simulink model "Gate_Harness"  (R2022b)
settings: Solver=VariableStepAuto  StartTime=0.0  StopTime=80.0  RelTol=1e-3
(part 2 of 2)

== stateflow chart Gate_Harness/Test Sequence ==
  settings: updateMethod=DISCRETE  sampleTime=0.2
  state Apertura_Chiusura_con_B1
    state INIT
      %% Initialize data outputs.
      p1 = true;
      p2 = false;
      start = false;
      b1 = false;
      b2 = false;
      b3 = false;
      verify(enable_green == false);
      verify(enable_yellow == false);
      verify(enable_red == false);
      verify(blink_green == false);
      verify(blink_yellow == false);
    state TURN_ON
      start = true;
    state CLOSE
      verify(enable_green == false);
      verify(enable_yellow == false);
      verify(enable_red == false);
      verify(blink_green == false);
      verify(blink_yellow == false);
    state PRESSED
      b1 = true;
    state RELEASED_BUTTON
      b1 = false;
    state OPENING_GATE
      p2 = true;
      verify(enable_green == false);
      verify(enable_yellow == false);
      verify(enable_red == false);
      verify(blink_green == false);
      verify(blink_yellow == true);
    state OPEN_GATE
      verify(enable_green == true);
      verify(enable_yellow == true);
      verify(enable_red == true);
      verify(blink_green == false);
      verify(blink_yellow == false);
    state PRESSED_AGAIN
      b1 = true;
    state RELEASED_BUTTON_AGAIN
      b1 = false;
    state CLOSING_GATE
      verify(enable_green == false);
      verify(enable_yellow == false);
      verify(enable_red == false);
      verify(blink_green == false);
      verify(blink_yellow == true);
    state ACTIVATE_P2
      p2 = false;
    state CLOSE_GATE
      verify(enable_green == false);
      verify(enable_yellow == false);
      verify(enable_red == false);
      verify(blink_green == false);
      verify(blink_yellow == false);
    state FINAL
    (default) -> Apertura_Chiusura_con_B1.INIT
    Apertura_Chiusura_con_B1.INIT -> Apertura_Chiusura_con_B1.TURN_ON : [
        | after(2, sec)
        | ]
    Apertura_Chiusura_con_B1.TURN_ON -> Apertura_Chiusura_con_B1.CLOSE : [
        | after(3, sec)
        | ]
    Apertura_Chiusura_con_B1.CLOSE -> Apertura_Chiusura_con_B1.PRESSED : [
        | after(2, sec)
        | ]
    Apertura_Chiusura_con_B1.PRESSED -> Apertura_Chiusura_con_B1.RELEASED_BUTTON : [
        | after(2, sec)
        | ]
    Apertura_Chiusura_con_B1.RELEASED_BUTTON -> Apertura_Chiusura_con_B1.OPENING_GATE : [
        | after(0.4, sec)
        | ]
    Apertura_Chiusura_con_B1.OPENING_GATE -> Apertura_Chiusura_con_B1.OPEN_GATE : [
        | after(10, sec)
        | ]
    Apertura_Chiusura_con_B1.OPEN_GATE -> Apertura_Chiusura_con_B1.PRESSED_AGAIN : [
        | after(4, sec)
        | ]
    Apertura_Chiusura_con_B1.PRESSED_AGAIN -> Apertura_Chiusura_con_B1.RELEASED_BUTTON_AGAIN : [
        | after(2, sec)
        | ]
    Apertura_Chiusura_con_B1.RELEASED_BUTTON_AGAIN -> Apertura_Chiusura_con_B1.CLOSING_GATE : [
        | after(0.4, sec)
        | ]
    Apertura_Chiusura_con_B1.CLOSING_GATE -> Apertura_Chiusura_con_B1.ACTIVATE_P2 : [
        | after(9.4, sec)
        | ]
    Apertura_Chiusura_con_B1.ACTIVATE_P2 -> Apertura_Chiusura_con_B1.CLOSE_GATE : [
        | after(1, sec)
        | ]
    Apertura_Chiusura_con_B1.CLOSE_GATE -> Apertura_Chiusura_con_B1.FINAL : [
        | after(6, sec)
        | ]
  state Chiusura_Automatica
    state INIT
      %% Initialize data outputs.
      p1 = true;
      p2 = false;
      start = false;
      b1 = false;
      b2 = false;
      b3 = false;
      verify(enable_green == false);
      verify(enable_yellow == false);
      verify(enable_red == false);
      verify(blink_green == false);
      verify(blink_yellow == false);
    state TURN_ON
      start = true;
    state CLOSE
      verify(enable_green == false);
      verify(enable_yellow == false);
      verify(enable_red == false);
      verify(blink_green == false);
      verify(blink_yellow == false);
    state PRESSED
      b1 = true;
    state RELEASED_BUTTON
      b1 = false;
    state OPENING_GATE
      p2 = true;
      verify(enable_green == false);
      verify(enable_yellow == false);
      verify(enable_red == false);
      verify(blink_green == false);
      verify(blink_yellow == true);
    state OPEN_GATE
      verify(enable_green == true);
      verify(enable_yellow == true);
      verify(enable_red == true);
      verify(blink_green == false);
      verify(blink_yellow == false);
    state CLOSING_GATE
      verify(enable_green == false);
      verify(enable_yellow == false);
      verify(enable_red == false);
      verify(blink_green == false);
      verify(blink_yellow == true);
    state ACTIVATE_P2
      p2 = false;
    state CLOSE_GATE
      verify(enable_green == false);
      verify(enable_yellow == false);
      verify(enable_red == false);
      verify(blink_green == false);
      verify(blink_yellow == false);
    state FINAL
    (default) -> Chiusura_Automatica.INIT
    Chiusura_Automatica.INIT -> Chiusura_Automatica.TURN_ON : [
        | after(2, sec)
        | ]
    Chiusura_Automatica.TURN_ON -> Chiusura_Automatica.CLOSE : [
        | after(3, sec)
        | ]
    Chiusura_Automatica.CLOSE -> Chiusura_Automatica.PRESSED : [
        | after(2, sec)
        | ]
    Chiusura_Automatica.PRESSED -> Chiusura_Automatica.RELEASED_BUTTON : [
        | after(2, sec)
        | ]
    Chiusura_Automatica.RELEASED_BUTTON -> Chiusura_Automatica.OPENING_GATE : [
        | after(0.4, sec)
        | ]
    Chiusura_Automatica.OPENING_GATE -> Chiusura_Automatica.OPEN_GATE : [
        | after(10, sec)
        | ]
    Chiusura_Automatica.OPEN_GATE -> Chiusura_Automatica.CLOSING_GATE : [
        | after(10, sec)
        | ]
    Chiusura_Automatica.CLOSING_GATE -> Chiusura_Automatica.ACTIVATE_P2 : [
        | after(9.4, sec)
        | ]
    Chiusura_Automatica.ACTIVATE_P2 -> Chiusura_Automatica.CLOSE_GATE : [
        | after(2, sec)
        | ]
    Chiusura_Automatica.CLOSE_GATE -> Chiusura_Automatica.FINAL : [
        | after(4, sec)
        | ]
  state Richiesta_Chiusura_durante_Apertura
    state INIT
      %% Initialize data outputs.
      p1 = true;
      p2 = false;
      start = false;
      b1 = false;
      b2 = false;
      b3 = false;
      verify(enable_green == false);
      verify(enable_yellow == false);
      verify(enable_red == false);
      verify(blink_green == false);
      verify(blink_yellow == false);
    state TURN_ON
      start = true;
    state CLOSE
      verify(enable_green == false);
      verify(enable_yellow == false);
      verify(enable_red == false);
      verify(blink_green == false);
      verify(blink_yellow == false);
    state PRESSED
      b1 = true;
    state RELEASED_BUTTON
      b1 = false;
    state OPENING_GATE
      p2 = true;
      verify(enable_green == false);
      verify(enable_yellow == false);
      verify(enable_red == false);
      verify(blink_green == false);
      verify(blink_yellow == true);
    state PRESSED_AGAIN
      b1 = true;
    state RELEASED_BUTTON_AGAIN
      b1 = false;
    state CLOSING_GATE
      verify(enable_green == false);
      verify(enable_yellow == false);
      verify(enable_red == false);
      verify(blink_green == false);
      verify(blink_yellow == true);
    state ACTIVATE_P2
      p2 = false;
    state CLOSE_GATE
      verify(enable_green == false);
      verify(enable_yellow == false);
      verify(enable_red == false);
      verify(blink_green == false);
      verify(blink_yellow == false);
    state FINAL
    (default) -> Richiesta_Chiusura_durante_Apertura.INIT
    Richiesta_Chiusura_durante_Apertura.INIT -> Richiesta_Chiusura_durante_Apertura.TURN_ON : [
        | after(2, sec)
        | ]
    Richiesta_Chiusura_durante_Apertura.TURN_ON -> Richiesta_Chiusura_durante_Apertura.CLOSE : [
        | after(3, sec)
        | ]
    Richiesta_Chiusura_durante_Apertura.CLOSE -> Richiesta_Chiusura_durante_Apertura.PRESSED : [
        | after(2, sec)
        | ]
    Richiesta_Chiusura_durante_Apertura.PRESSED -> Richiesta_Chiusura_durante_Apertura.RELEASED_BUTTON : [
        | after(2, sec)
        | ]
    Richiesta_Chiusura_durante_Apertura.RELEASED_BUTTON -> Richiesta_Chiusura_durante_Apertura.OPENING_GATE : [
        | after(0.4, sec)
        | ]
    Richiesta_Chiusura_durante_Apertura.OPENING_GATE -> Richiesta_Chiusura_durante_Apertura.PRESSED_AGAIN : [
        | after(3, sec)
        | ]
    Richiesta_Chiusura_durante_Apertura.PRESSED_AGAIN -> Richiesta_Chiusura_durante_Apertura.RELEASED_BUTTON_AGAIN : [
        | after(2, sec)
        | ]
    Richiesta_Chiusura_durante_Apertura.RELEASED_BUTTON_AGAIN -> Richiesta_Chiusura_durante_Apertura.CLOSING_GATE : [
        | after(0.4, sec)
        | ]
    Richiesta_Chiusura_durante_Apertura.CLOSING_GATE -> Richiesta_Chiusura_durante_Apertura.ACTIVATE_P2 : [
        | after(9.4, sec)
        | ]
    Richiesta_Chiusura_durante_Apertura.ACTIVATE_P2 -> Richiesta_Chiusura_durante_Apertura.CLOSE_GATE : [
        | after(1, sec)
        | ]
    Richiesta_Chiusura_durante_Apertura.CLOSE_GATE -> Richiesta_Chiusura_durante_Apertura.FINAL : [
        | after(6, sec)
        | ]
  state Richiesta_Apertura_durante_Chiusura
    state INIT
      %% Initialize data outputs.
      p1 = true;
      p2 = true;
      start = false;
      b1 = false;
      b2 = false;
      b3 = false;
      verify(enable_green == false);
      verify(enable_yellow == false);
      verify(enable_red == false);
      verify(blink_green == false);
      verify(blink_yellow == false);
    state TURN_ON
      start = true;
    state CLOSING_GATE
      verify(enable_green == false);
      verify(enable_yellow == false);
      verify(enable_red == false);
      verify(blink_green == false);
      verify(blink_yellow == true);
    state B1_PRESSED
      b1 = true;
    state B1_RELEASED
      b1 = false;
    state OPENING_GATE
      verify(enable_green == false);
      verify(enable_yellow == false);
      verify(enable_red == false);
      verify(blink_green == false);
      verify(blink_yellow == true);
    state FINAL
      start = false;
    (default) -> Richiesta_Apertura_durante_Chiusura.INIT
    Richiesta_Apertura_durante_Chiusura.INIT -> Richiesta_Apertura_durante_Chiusura.TURN_ON : [
        | after(2, sec)
        | ]
    Richiesta_Apertura_durante_Chiusura.CLOSING_GATE -> Richiesta_Apertura_durante_Chiusura.B1_PRESSED : [
        | after(4, sec)
        | ]
    Richiesta_Apertura_durante_Chiusura.B1_PRESSED -> Richiesta_Apertura_durante_Chiusura.B1_RELEASED : [
        | after(2, sec)
        | ]
    Richiesta_Apertura_durante_Chiusura.B1_RELEASED -> Richiesta_Apertura_durante_Chiusura.OPENING_GATE : [
        | after(0.4, sec)
        | ]
    Richiesta_Apertura_durante_Chiusura.OPENING_GATE -> Richiesta_Apertura_durante_Chiusura.FINAL : [
        | after(4, sec)
        | ]
    Richiesta_Apertura_durante_Chiusura.TURN_ON -> Richiesta_Apertura_durante_Chiusura.CLOSING_GATE : [
        | after(3, sec)
        | ]
  state Incremento_Tempo_Lavoro
    state INIT
      %% Initialize data outputs.
      p1 = true;
      p2 = false;
      start = false;
      b1 = false;
      b2 = false;
      b3 = false;
      n = 0;
      verify(enable_green == false);
      verify(enable_yellow == false);
      verify(enable_red == false);
      verify(blink_green == false);
      verify(blink_yellow == false);
    state TURN_ON
      start = true;
    state CLOSE
      verify(enable_green == false);
      verify(enable_yellow == false);
      verify(enable_red == false);
      verify(blink_green == false);
      verify(blink_yellow == false);
    state B3
      settings: description=|
          | In questa transizione
          | il valore può essere
          | modificato per decidere
          | quante volte deve
          | essere incrementato
          | il tempo di lavoro. n=0
          | indica nessun incremento,
          | n=11 porta il tempo a
          | 120 secondi, n=12 lo
          | riporta a 10.
      state B3_PRESSED
        b3 = true;
      state B3_RELEASED
        b3 = false;
      state B3_INTERMEDIATE
        n = n +1;
      (default) -> B3_PRESSED
      (junction 326) -> B3_PRESSED
      B3_PRESSED -> B3_RELEASED : [
          | after(1, sec)
          | ]
      B3_RELEASED -> B3_INTERMEDIATE : [
          | after(1, sec)
          | ]
      B3_INTERMEDIATE -> (junction 328) : [
          | true
          | ]
      (junction 328) -> (junction 326)
    state B1_PRESSED
      b1 = true;
    state B1_RELEASED
      b1 = false;
    state OPENING_GATE
      p2 = true;
      verify(enable_green == false);
      verify(enable_yellow == false);
      verify(enable_red == false);
      verify(blink_green == false);
      verify(blink_yellow == true);
      settings: description=|
          | Questa transizione
          | permette di aspettare
          | un tempo pari al tempo
          | di lavoro in base a
          | quante volte è stato
          | premuto B3 in
          | precedenza
    state OPEN_GATE
      verify(enable_green == true);
      verify(enable_yellow == true);
      verify(enable_red == true);
      verify(blink_green == false);
      verify(blink_yellow == false);
    state FINAL
      p2 = false;
    (default) -> Incremento_Tempo_Lavoro.INIT
    Incremento_Tempo_Lavoro.INIT -> Incremento_Tempo_Lavoro.TURN_ON : [
        | after(2, sec)
        | ]
    Incremento_Tempo_Lavoro.TURN_ON -> Incremento_Tempo_Lavoro.CLOSE : [
        | after(3, sec)
        | ]
    Incremento_Tempo_Lavoro.CLOSE -> B3 : [
        | after(2, sec)
        | ]
    Incremento_Tempo_Lavoro.B1_PRESSED -> Incremento_Tempo_Lavoro.B1_RELEASED : [
        | after(2, sec)
        | ]
    Incremento_Tempo_Lavoro.B1_RELEASED -> Incremento_Tempo_Lavoro.OPENING_GATE : [
        | after(0.4, sec)
        | ]
    Incremento_Tempo_Lavoro.OPENING_GATE -> Incremento_Tempo_Lavoro.OPEN_GATE : [
        | after(mod(n*INCREMENT, MAX) + INCREMENT, sec)
        | ]
    Incremento_Tempo_Lavoro.OPEN_GATE -> Incremento_Tempo_Lavoro.FINAL : [
        | after(5, sec)
        | ]
    B3 -> Incremento_Tempo_Lavoro.B1_PRESSED : [
        | n == 12
        | ]
  state Incremento_Tempo_Chiusura_Automatica
    state INIT
      %% Initialize data outputs.
      p1 = true;
      p2 = false;
      start = false;
      b1 = false;
      b2 = false;
      b3 = false;
      n = 0;
      verify(enable_green == false);
      verify(enable_yellow == false);
      verify(enable_red == false);
      verify(blink_green == false);
      verify(blink_yellow == false);
    state TURN_ON
      start = true;
    state CLOSE
      verify(enable_green == false);
      verify(enable_yellow == false);
      verify(enable_red == false);
      verify(blink_green == false);
      verify(blink_yellow == false);
    state B2
      settings: description=|
          | In questa transizione
          | il valore può essere
          | modificato per decidere
          | quante volte deve
          | essere incrementato
          | il tempo di chiusura
          | automatica. n=0
          | indica nessun incremento,
          | n=11 porta il tempo a
          | 120 secondi, n=12 lo
          | riporta a 10.
      state B2_PRESSED
        b2 = true;
      state B2_RELEASED
        b2 = false;
      state B2_INTERMEDIATE
        n = n+1;
      B2_INTERMEDIATE -> (junction 584) : [
          | true
          | ]
      (default) -> B2_PRESSED
      (junction 582) -> B2_PRESSED
      B2_PRESSED -> B2_RELEASED : [
          | after(1, sec)
          | ]
      B2_RELEASED -> B2_INTERMEDIATE : [
          | after(1, sec)
          | ]
      (junction 584) -> (junction 582)
    state B1_PRESSED
      b1 = true;
    state B1_RELEASED
      b1 = false;
    state OPENING_GATE
      p2 = true;
      verify(enable_green == false);
      verify(enable_yellow == false);
      verify(enable_red == false);
      verify(blink_green == false);
      verify(blink_yellow == true);
    state OPEN_GATE
      verify(enable_green == true);
      verify(enable_yellow == true);
      verify(enable_red == true);
      verify(blink_green == false);
      verify(blink_yellow == false);
      settings: description=|
          | Questa transizione
          | permette di aspettare
          | un tempo pari al tempo
          | di chiusura automatica
          | in base a quante volte
          | è stato premuto B2 in
          | precedenza
    state CLOSING_GATE
      verify(enable_green == false);
      verify(enable_yellow == false);
      verify(enable_red == false);
      verify(blink_green == false);
      verify(blink_yellow == true);
    state CLOSE_GATE
      p2 = false;
      verify(enable_green == false);
      verify(enable_yellow == false);
      verify(enable_red == false);
      verify(blink_green == false);
      verify(blink_yellow == false);
    state FINAL
    (default) -> Incremento_Tempo_Chiusura_Automatica.INIT
    Incremento_Tempo_Chiusura_Automatica.INIT -> Incremento_Tempo_Chiusura_Automatica.TURN_ON : [
        | after(2, sec)
        | ]
    Incremento_Tempo_Chiusura_Automatica.TURN_ON -> Incremento_Tempo_Chiusura_Automatica.CLOSE : [
        | after(3, sec)
        | ]
    Incremento_Tempo_Chiusura_Automatica.B1_PRESSED -> Incremento_Tempo_Chiusura_Automatica.B1_RELEASED : [
        | after(2, sec)
        | ]
    Incremento_Tempo_Chiusura_Automatica.B1_RELEASED -> Incremento_Tempo_Chiusura_Automatica.OPENING_GATE : [
        | after(0.4, sec)
        | ]
    Incremento_Tempo_Chiusura_Automatica.OPENING_GATE -> Incremento_Tempo_Chiusura_Automatica.OPEN_GATE : [
        | after(10, sec)
        | ]
    Incremento_Tempo_Chiusura_Automatica.OPEN_GATE -> Incremento_Tempo_Chiusura_Automatica.CLOSING_GATE : [
        | after(mod(n*INCREMENT, MAX) + INCREMENT, sec)
        | ]
    Incremento_Tempo_Chiusura_Automatica.CLOSING_GATE -> Incremento_Tempo_Chiusura_Automatica.CLOSE_GATE : [
        | after(10, sec)
        | ]
    Incremento_Tempo_Chiusura_Automatica.CLOSE_GATE -> Incremento_Tempo_Chiusura_Automatica.FINAL : [
        | after(4, sec)
        | ]
    B2 -> Incremento_Tempo_Chiusura_Automatica.B1_PRESSED : [
        | n == 12
        | ]
    Incremento_Tempo_Chiusura_Automatica.CLOSE -> B2 : [
        | after(2, sec)
        | ]
  state Gestione_Situazione_Errore
    state INIT
      %% Initialize data outputs.
      p1 = true;
      p2 = true;
      start = false;
      b1 = false;
      b2 = false;
      b3 = false;
      verify(enable_green == false);
      verify(enable_yellow == false);
      verify(enable_red == false);
      verify(blink_green == false);
      verify(blink_yellow == false);
      settings: description=|
          | Il cancello parte da
          | spento e aperto.
    state TURN_ON
      start = true;
    state CLOSING_GATE
      verify(enable_green == false);
      verify(enable_yellow == false);
      verify(enable_red == false);
      verify(blink_green == false);
      verify(blink_yellow == true);
    state STOP_GATE
      verify(enable_green == false);
      verify(enable_yellow == false);
      verify(enable_red == false);
      verify(blink_green == false);
      verify(blink_yellow == false);
    state ERROR_GATE
      verify(enable_green == false);
      verify(enable_yellow == false);
      verify(enable_red == true);
      verify(blink_green == false);
      verify(blink_yellow == false);
    state ACTIVATE_P2
      p2 = false;
    state CLOSE_GATE
      verify(enable_green == false);
      verify(enable_yellow == false);
      verify(enable_red == false);
      verify(blink_green == false);
      verify(blink_yellow == false);
    state FINAL
    (default) -> Gestione_Situazione_Errore.INIT
    Gestione_Situazione_Errore.INIT -> Gestione_Situazione_Errore.TURN_ON : [
        | after(2, sec)
        | ]
    Gestione_Situazione_Errore.TURN_ON -> Gestione_Situazione_Errore.CLOSING_GATE : [
        | after(0.4, sec)
        | ]
    Gestione_Situazione_Errore.CLOSING_GATE -> Gestione_Situazione_Errore.STOP_GATE : [
        | after(10, sec)
        | ]
    Gestione_Situazione_Errore.ERROR_GATE -> Gestione_Situazione_Errore.ACTIVATE_P2 : [
        | after(4, sec)
        | ]
    Gestione_Situazione_Errore.ACTIVATE_P2 -> Gestione_Situazione_Errore.CLOSE_GATE : [
        | after(1, sec)
        | ]
    Gestione_Situazione_Errore.CLOSE_GATE -> Gestione_Situazione_Errore.FINAL : [
        | after(4, sec)
        | ]
    Gestione_Situazione_Errore.STOP_GATE -> Gestione_Situazione_Errore.ERROR_GATE : [
        | after(10, sec)
        | ]
  state Stato_di_Blocco
    state INIT
      %% Initialize data outputs.
      p1 = true;
      p2 = true;
      start = false;
      b1 = false;
      b2 = false;
      b3 = false;
      verify(enable_green == false);
      verify(enable_yellow == false);
      verify(enable_red == false);
      verify(blink_green == false);
      verify(blink_yellow == false);
      settings: description=|
          | Il cancello parte da
          | spento e aperto.
    state TURN_ON
      start = true;
    state CLOSING_GATE
      verify(enable_green == false);
      verify(enable_yellow == false);
      verify(enable_red == false);
      verify(blink_green == false);
      verify(blink_yellow == true);
    state STOP_GATE
      verify(enable_green == false);
      verify(enable_yellow == false);
      verify(enable_red == false);
      verify(blink_green == false);
      verify(blink_yellow == false);
    state B1_PRESSED
      b1 = true;
    state B1_RELEASED
      b1 = false;
    state IGNORE_COMMAND
      verify(enable_green == false);
      verify(enable_yellow == false);
      verify(enable_red == false);
      verify(blink_green == false);
      verify(blink_yellow == false);
      settings: description=|
          | Controllo che quando
          | si trova nello stato
          | STOP_SYSTEM, il
          | cancello ignora input
          | come la pressione di
          | B1. Verifico quindi che
          | siamo ancora nello
          | stesso stato.
    state ERROR_GATE
      verify(enable_green == false);
      verify(enable_yellow == false);
      verify(enable_red == true);
      verify(blink_green == false);
      verify(blink_yellow == false);
    state FINAL
    (default) -> Stato_di_Blocco.INIT
    Stato_di_Blocco.INIT -> Stato_di_Blocco.TURN_ON : [
        | after(2, sec)
        | ]
    Stato_di_Blocco.TURN_ON -> Stato_di_Blocco.CLOSING_GATE : [
        | after(0.4, sec)
        | ]
    Stato_di_Blocco.CLOSING_GATE -> Stato_di_Blocco.STOP_GATE : [
        | after(10, sec)
        | ]
    Stato_di_Blocco.STOP_GATE -> Stato_di_Blocco.B1_PRESSED : [
        | after(3, sec)
        | ]
    Stato_di_Blocco.B1_PRESSED -> Stato_di_Blocco.B1_RELEASED : [
        | after(2, sec)
        | ]
    Stato_di_Blocco.B1_RELEASED -> Stato_di_Blocco.IGNORE_COMMAND : [
        | after(2, sec)
        | ]
    Stato_di_Blocco.IGNORE_COMMAND -> Stato_di_Blocco.ERROR_GATE : [
        | after(3, sec)
        | ]
    Stato_di_Blocco.ERROR_GATE -> Stato_di_Blocco.FINAL : [
        | after(4, sec)
        | ]
  state Stato_di_Errore
    state INIT
      %% Initialize data outputs.
      p1 = true;
      p2 = true;
      start = false;
      b1 = false;
      b2 = false;
      b3 = false;
      verify(enable_green == false);
      verify(enable_yellow == false);
      verify(enable_red == false);
      verify(blink_green == false);
      verify(blink_yellow == false);
      settings: description=|
          | Il cancello parte da
          | spento e aperto.
    state TURN_ON
      start = true;
    state CLOSING_GATE
      verify(enable_green == false);
      verify(enable_yellow == false);
      verify(enable_red == false);
      verify(blink_green == false);
      verify(blink_yellow == true);
    state STOP_GATE
      verify(enable_green == false);
      verify(enable_yellow == false);
      verify(enable_red == false);
      verify(blink_green == false);
      verify(blink_yellow == false);
    state ERROR_GATE
      verify(enable_green == false);
      verify(enable_yellow == false);
      verify(enable_red == true);
      verify(blink_green == false);
      verify(blink_yellow == false);
    state B1_PRESSED
      b1 = true;
    state B1_RELEASED
      b1 = false;
    state IGNORE_COMMAND
      verify(enable_green == false);
      verify(enable_yellow == false);
      verify(enable_red == true);
      verify(blink_green == false);
      verify(blink_yellow == false);
      settings: description=|
          | Controllo che quando
          | si trova nello stato
          | ERROR_STATE, il
          | cancello ignora input
          | come la pressione di
          | B1. Verifico quindi che
          | siamo ancora nello
          | stesso stato.
    state FINAL
    (default) -> Stato_di_Errore.INIT
    Stato_di_Errore.INIT -> Stato_di_Errore.TURN_ON : [
        | after(2, sec)
        | ]
    Stato_di_Errore.TURN_ON -> Stato_di_Errore.CLOSING_GATE : [
        | after(0.4, sec)
        | ]
    Stato_di_Errore.CLOSING_GATE -> Stato_di_Errore.STOP_GATE : [
        | after(10, sec)
        | ]
    Stato_di_Errore.STOP_GATE -> Stato_di_Errore.ERROR_GATE : [
        | after(10, sec)
        | ]
    Stato_di_Errore.ERROR_GATE -> Stato_di_Errore.B1_PRESSED : [
        | after(4, sec)
        | ]
    Stato_di_Errore.B1_PRESSED -> Stato_di_Errore.B1_RELEASED : [
        | after(2, sec)
        | ]
    Stato_di_Errore.B1_RELEASED -> Stato_di_Errore.IGNORE_COMMAND : [
        | after(2, sec)
        | ]
    Stato_di_Errore.IGNORE_COMMAND -> Stato_di_Errore.FINAL : [
        | after(3, sec)
        | ]
  state Rilevamento_Ostacolo_in_Chiusura
    state INIT
      %% Initialize data outputs.
      p1 = true;
      p2 = true;
      start = false;
      b1 = false;
      b2 = false;
      b3 = false;
      verify(enable_green == false);
      verify(enable_yellow == false);
      verify(enable_red == false);
      verify(blink_green == false);
      verify(blink_yellow == false);
    state TURN_ON
      start = true;
    state CLOSING_GATE
      verify(enable_green == false);
      verify(enable_yellow == false);
      verify(enable_red == false);
      verify(blink_green == false);
      verify(blink_yellow == true);
    state ACTIVATE_P1
      p1 = false;
    state OPENING_GATE
      verify(enable_green == false);
      verify(enable_yellow == false);
      verify(enable_red == false);
      verify(blink_green == false);
      verify(blink_yellow == true);
    state OPEN_GATE
      verify(enable_green == true);
      verify(enable_yellow == true);
      verify(enable_red == true);
      verify(blink_green == false);
      verify(blink_yellow == false);
    state FINAL
    (default) -> Rilevamento_Ostacolo_in_Chiusura.INIT
    Rilevamento_Ostacolo_in_Chiusura.INIT -> Rilevamento_Ostacolo_in_Chiusura.TURN_ON : [
        | after(2, sec)
        | ]
    Rilevamento_Ostacolo_in_Chiusura.TURN_ON -> Rilevamento_Ostacolo_in_Chiusura.CLOSING_GATE : [
        | after(0.4, sec)
        | ]
    Rilevamento_Ostacolo_in_Chiusura.CLOSING_GATE -> Rilevamento_Ostacolo_in_Chiusura.ACTIVATE_P1 : [
        | after(2, sec)
        | ]
    Rilevamento_Ostacolo_in_Chiusura.ACTIVATE_P1 -> Rilevamento_Ostacolo_in_Chiusura.OPENING_GATE : [
        | after(0.4, sec)
        | ]
    Rilevamento_Ostacolo_in_Chiusura.OPENING_GATE -> Rilevamento_Ostacolo_in_Chiusura.OPEN_GATE : [
        | after(10, sec)
        | ]
    Rilevamento_Ostacolo_in_Chiusura.OPEN_GATE -> Rilevamento_Ostacolo_in_Chiusura.FINAL : [
        | after(2, sec)
        | ]
  state RIlevamento_Ostacolo_in_Apertura
    state INIT
      %% Initialize data outputs.
      p1 = true;
      p2 = false;
      start = false;
      b1 = false;
      b2 = false;
      b3 = false;
      verify(enable_green == false);
      verify(enable_yellow == false);
      verify(enable_red == false);
      verify(blink_green == false);
      verify(blink_yellow == false);
    state TURN_ON
      start = true;
    state CLOSE_GATE
      verify(enable_green == false);
      verify(enable_yellow == false);
      verify(enable_red == false);
      verify(blink_green == false);
      verify(blink_yellow == false);
    state B1_PRESSED
      b1 = true;
    state B1_RELEASED
      b1 = false;
    state OPENING_GATE
      verify(enable_green == false);
      verify(enable_yellow == false);
      verify(enable_red == false);
      verify(blink_green == false);
      verify(blink_yellow == true);
    state ACTIVATE_P1
      p1 = false;
    state B1_PRESSED_AGAIN
      b1 = true;
    state B1_RELEASED_AGAIN
      b1 = false;
    state IGNORE_COMMAND
      verify(enable_green == false);
      verify(enable_yellow == false);
      verify(enable_red == false);
      verify(blink_green == false);
      verify(blink_yellow == true);
    state OPEN_GATE
      verify(enable_green == true);
      verify(enable_yellow == true);
      verify(enable_red == true);
      verify(blink_green == false);
      verify(blink_yellow == false);
    state FINAL
    (default) -> RIlevamento_Ostacolo_in_Apertura.INIT
    RIlevamento_Ostacolo_in_Apertura.INIT -> RIlevamento_Ostacolo_in_Apertura.TURN_ON : [
        | after(2, sec)
        | ]
    RIlevamento_Ostacolo_in_Apertura.TURN_ON -> RIlevamento_Ostacolo_in_Apertura.CLOSE_GATE : [
        | after(2, sec)
        | ]
    RIlevamento_Ostacolo_in_Apertura.CLOSE_GATE -> RIlevamento_Ostacolo_in_Apertura.B1_PRESSED : [
        | after(2, sec)
        | ]
    RIlevamento_Ostacolo_in_Apertura.B1_PRESSED -> RIlevamento_Ostacolo_in_Apertura.B1_RELEASED : [
        | after(2, sec)
        | ]
    RIlevamento_Ostacolo_in_Apertura.B1_RELEASED -> RIlevamento_Ostacolo_in_Apertura.OPENING_GATE : [
        | after(0.4, sec)
        | ]
    RIlevamento_Ostacolo_in_Apertura.OPENING_GATE -> RIlevamento_Ostacolo_in_Apertura.ACTIVATE_P1 : [
        | after(2, sec)
        | ]
    RIlevamento_Ostacolo_in_Apertura.ACTIVATE_P1 -> RIlevamento_Ostacolo_in_Apertura.B1_PRESSED_AGAIN : [
        | after(0.4, sec)
        | ]
    RIlevamento_Ostacolo_in_Apertura.B1_PRESSED_AGAIN -> B1_RELEASED_AGAIN : [
        | after(2, sec)
        | ]
    B1_RELEASED_AGAIN -> RIlevamento_Ostacolo_in_Apertura.IGNORE_COMMAND : [
        | after(0.4, sec)
        | ]
    RIlevamento_Ostacolo_in_Apertura.IGNORE_COMMAND -> RIlevamento_Ostacolo_in_Apertura.OPEN_GATE : [
        | after(5.4, sec)
        | ]
    RIlevamento_Ostacolo_in_Apertura.OPEN_GATE -> RIlevamento_Ostacolo_in_Apertura.FINAL : [
        | after(6, sec)
        | ]
  state Interruzione_Tempo_Chiusura_Automatica_con_Ostacoli
    state INIT
      %% Initialize data outputs.
      p1 = true;
      p2 = false;
      start = false;
      b1 = false;
      b2 = false;
      b3 = false;
      verify(enable_green == false);
      verify(enable_yellow == false);
      verify(enable_red == false);
      verify(blink_green == false);
      verify(blink_yellow == false);
      settings: description=|
          | Questo test serve a
          | controllare che se il
          | cancello è aperto e
          | viene rilevato un
          | ostacolo, non viene
          | considerato il tempo
          | di chiusura automatica
          | fin quando non viene
          | rimosso l'ostacolo.
    state TURN_ON
      start = true;
    state CLOSE
      verify(enable_green == false);
      verify(enable_yellow == false);
      verify(enable_red == false);
      verify(blink_green == false);
      verify(blink_yellow == false);
    state B1_PRESSED1
      b1 = true;
    state B1_RELEASED_BUTTON
      b1 = false;
    state OPENING_GATE
      p2 = true;
      verify(enable_green == false);
      verify(enable_yellow == false);
      verify(enable_red == false);
      verify(blink_green == false);
      verify(blink_yellow == true);
    state OPEN_GATE
      verify(enable_green == true);
      verify(enable_yellow == true);
      verify(enable_red == true);
      verify(blink_green == false);
      verify(blink_yellow == false);
    state ACTIVATE_P1
      p1 = false;
    state DEACTIVATE_P1
      p1 = true;
    state CHECK_OPEN_GATE
      verify(enable_green == true);
      verify(enable_yellow == true);
      verify(enable_red == true);
      verify(blink_green == false);
      verify(blink_yellow == false);
    state CLOSING_GATE
      verify(enable_green == false);
      verify(enable_yellow == false);
      verify(enable_red == false);
      verify(blink_green == false);
      verify(blink_yellow == true);
      settings: description=|
          | A questo punto sono
          | passati più di 10
          | secondi da quando il
          | cancello si è aperto, il
          | che conferma che il
          | tempo di chiusura
          | automatica si sia
          | temporaneamente
          | interrotto.
    state FINAL
      p2 = false;
    (default) -> Interruzione_Tempo_Chiusura_Automatica_con_Ostacoli.INIT
    Interruzione_Tempo_Chiusura_Automatica_con_Ostacoli.INIT -> Interruzione_Tempo_Chiusura_Automatica_con_Ostacoli.TURN_ON : [
        | after(2, sec)
        | ]
    Interruzione_Tempo_Chiusura_Automatica_con_Ostacoli.TURN_ON -> Interruzione_Tempo_Chiusura_Automatica_con_Ostacoli.CLOSE : [
        | after(3, sec)
        | ]
    Interruzione_Tempo_Chiusura_Automatica_con_Ostacoli.CLOSE -> B1_PRESSED1 : [
        | after(2, sec)
        | ]
    B1_PRESSED1 -> Interruzione_Tempo_Chiusura_Automatica_con_Ostacoli.B1_RELEASED_BUTTON : [
        | after(2, sec)
        | ]
    Interruzione_Tempo_Chiusura_Automatica_con_Ostacoli.B1_RELEASED_BUTTON -> Interruzione_Tempo_Chiusura_Automatica_con_Ostacoli.OPENING_GATE : [
        | after(0.4, sec)
        | ]
    Interruzione_Tempo_Chiusura_Automatica_con_Ostacoli.OPENING_GATE -> Interruzione_Tempo_Chiusura_Automatica_con_Ostacoli.OPEN_GATE : [
        | after(10, sec)
        | ]
    Interruzione_Tempo_Chiusura_Automatica_con_Ostacoli.OPEN_GATE -> Interruzione_Tempo_Chiusura_Automatica_con_Ostacoli.ACTIVATE_P1 : [
        | after(4, sec)
        | ]
    Interruzione_Tempo_Chiusura_Automatica_con_Ostacoli.ACTIVATE_P1 -> Interruzione_Tempo_Chiusura_Automatica_con_Ostacoli.DEACTIVATE_P1 : [
        | after(2, sec)
        | ]
    Interruzione_Tempo_Chiusura_Automatica_con_Ostacoli.DEACTIVATE_P1 -> CHECK_OPEN_GATE : [
        | after(0.4, sec)
        | ]
    CHECK_OPEN_GATE -> Interruzione_Tempo_Chiusura_Automatica_con_Ostacoli.CLOSING_GATE : [
        | after(10, sec)
        | ]
    Interruzione_Tempo_Chiusura_Automatica_con_Ostacoli.CLOSING_GATE -> Interruzione_Tempo_Chiusura_Automatica_con_Ostacoli.FINAL : [
        | after(9.4, sec)
        | ]
  state Interruzione_LED_Verde_in_Aperto_P1_Disattivo
    state INIT
      %% Initialize data outputs.
      p1 = true;
      p2 = false;
      start = false;
      b1 = false;
      b2 = false;
      b3 = false;
      verify(enable_green == false);
      verify(enable_yellow == false);
      verify(enable_red == false);
      verify(blink_green == false);
      verify(blink_yellow == false);
    state TURN_ON
      start = true;
    state CLOSE
      verify(enable_green == false);
      verify(enable_yellow == false);
      verify(enable_red == false);
      verify(blink_green == false);
      verify(blink_yellow == false);
    state PRESSED
      b1 = true;
    state RELEASED_BUTTON
      b1 = false;
    state OPENING_GATE
      p2 = true;
      verify(enable_green == false);
      verify(enable_yellow == false);
      verify(enable_red == false);
      verify(blink_green == false);
      verify(blink_yellow == true);
    state OPEN_GATE
      verify(enable_green == true);
      verify(enable_yellow == true);
      verify(enable_red == true);
      verify(blink_green == false);
      verify(blink_yellow == false);
    state ACTIVATE_P1
      p1 = false;
    state B1_PRESSED
      b1 = true;
    state B1_RELEASED_BUTTON
      b1 = false;
    state IGNORE_COMMAND
      verify(enable_green == false);
      verify(enable_yellow == false);
      verify(enable_red == false);
      verify(blink_green == true);
      verify(blink_yellow == false);
    state DEACTIVATE_P1
      p1 = true;
    state VERIFY_DEACTIVATION
      verify(enable_green == true);
      verify(enable_yellow == true);
      verify(enable_red == true);
      verify(blink_green == false);
      verify(blink_yellow == false);
    state FINAL
      p2 = false;
    (default) -> Interruzione_LED_Verde_in_Aperto_P1_Disattivo.INIT
    Interruzione_LED_Verde_in_Aperto_P1_Disattivo.INIT -> Interruzione_LED_Verde_in_Aperto_P1_Disattivo.TURN_ON : [
        | after(2, sec)
        | ]
    Interruzione_LED_Verde_in_Aperto_P1_Disattivo.TURN_ON -> Interruzione_LED_Verde_in_Aperto_P1_Disattivo.CLOSE : [
        | after(3, sec)
        | ]
    Interruzione_LED_Verde_in_Aperto_P1_Disattivo.CLOSE -> Interruzione_LED_Verde_in_Aperto_P1_Disattivo.PRESSED : [
        | after(2, sec)
        | ]
    Interruzione_LED_Verde_in_Aperto_P1_Disattivo.PRESSED -> Interruzione_LED_Verde_in_Aperto_P1_Disattivo.RELEASED_BUTTON : [
        | after(2, sec)
        | ]
    Interruzione_LED_Verde_in_Aperto_P1_Disattivo.RELEASED_BUTTON -> Interruzione_LED_Verde_in_Aperto_P1_Disattivo.OPENING_GATE : [
        | after(0.4, sec)
        | ]
    Interruzione_LED_Verde_in_Aperto_P1_Disattivo.OPENING_GATE -> Interruzione_LED_Verde_in_Aperto_P1_Disattivo.OPEN_GATE : [
        | after(10, sec)
        | ]
    Interruzione_LED_Verde_in_Aperto_P1_Disattivo.OPEN_GATE -> Interruzione_LED_Verde_in_Aperto_P1_Disattivo.ACTIVATE_P1 : [
        | after(2, sec)
        | ]
    Interruzione_LED_Verde_in_Aperto_P1_Disattivo.ACTIVATE_P1 -> Interruzione_LED_Verde_in_Aperto_P1_Disattivo.B1_PRESSED : [
        | after(0.4, sec)
        | ]
    Interruzione_LED_Verde_in_Aperto_P1_Disattivo.B1_PRESSED -> Interruzione_LED_Verde_in_Aperto_P1_Disattivo.B1_RELEASED_BUTTON : [
        | after(2, sec)
        | ]
    Interruzione_LED_Verde_in_Aperto_P1_Disattivo.B1_RELEASED_BUTTON -> Interruzione_LED_Verde_in_Aperto_P1_Disattivo.IGNORE_COMMAND : [
        | after(0.4, sec)
        | ]
    Interruzione_LED_Verde_in_Aperto_P1_Disattivo.IGNORE_COMMAND -> Interruzione_LED_Verde_in_Aperto_P1_Disattivo.DEACTIVATE_P1 : [
        | after(1, sec)
        | ]
    Interruzione_LED_Verde_in_Aperto_P1_Disattivo.DEACTIVATE_P1 -> Interruzione_LED_Verde_in_Aperto_P1_Disattivo.VERIFY_DEACTIVATION : [
        | after(0.4, sec)
        | ]
    Interruzione_LED_Verde_in_Aperto_P1_Disattivo.VERIFY_DEACTIVATION -> Interruzione_LED_Verde_in_Aperto_P1_Disattivo.FINAL : [
        | after(1, sec)
        | ]
  state Interruzione_LED_Verde_in_Chiuso_P1_Disattivo
    state INIT
      %% Initialize data outputs.
      p1 = true;
      p2 = false;
      start = false;
      b1 = false;
      b2 = false;
      b3 = false;
      verify(enable_green == false);
      verify(enable_yellow == false);
      verify(enable_red == false);
      verify(blink_green == false);
      verify(blink_yellow == false);
    state TURN_ON
      start = true;
    state CLOSE
      verify(enable_green == false);
      verify(enable_yellow == false);
      verify(enable_red == false);
      verify(blink_green == false);
      verify(blink_yellow == false);
    state ACTIVATE_P1
      p1 = false;
    state PRESSED
      b1 = true;
    state RELEASED_BUTTON
      b1 = false;
    state IGNORE_COMMAND
      verify(enable_green == false);
      verify(enable_yellow == false);
      verify(enable_red == false);
      verify(blink_green == true);
      verify(blink_yellow == false);
    state DEACTIVATE_P1
      p1 = true;
    state VERIFY_DEACTIVATION
      verify(enable_green == false);
      verify(enable_yellow == false);
      verify(enable_red == false);
      verify(blink_green == false);
      verify(blink_yellow == false);
    state FINAL
    (default) -> Interruzione_LED_Verde_in_Chiuso_P1_Disattivo.INIT
    Interruzione_LED_Verde_in_Chiuso_P1_Disattivo.INIT -> Interruzione_LED_Verde_in_Chiuso_P1_Disattivo.TURN_ON : [
        | after(2, sec)
        | ]
    Interruzione_LED_Verde_in_Chiuso_P1_Disattivo.TURN_ON -> Interruzione_LED_Verde_in_Chiuso_P1_Disattivo.CLOSE : [
        | after(3, sec)
        | ]
    Interruzione_LED_Verde_in_Chiuso_P1_Disattivo.CLOSE -> Interruzione_LED_Verde_in_Chiuso_P1_Disattivo.ACTIVATE_P1 : [
        | after(2, sec)
        | ]
    Interruzione_LED_Verde_in_Chiuso_P1_Disattivo.ACTIVATE_P1 -> Interruzione_LED_Verde_in_Chiuso_P1_Disattivo.PRESSED : [
        | after(0.4, sec)
        | ]
    Interruzione_LED_Verde_in_Chiuso_P1_Disattivo.PRESSED -> Interruzione_LED_Verde_in_Chiuso_P1_Disattivo.RELEASED_BUTTON : [
        | after(2, sec)
        | ]
    Interruzione_LED_Verde_in_Chiuso_P1_Disattivo.RELEASED_BUTTON -> Interruzione_LED_Verde_in_Chiuso_P1_Disattivo.IGNORE_COMMAND : [
        | after(0.4, sec)
        | ]
    Interruzione_LED_Verde_in_Chiuso_P1_Disattivo.IGNORE_COMMAND -> Interruzione_LED_Verde_in_Chiuso_P1_Disattivo.DEACTIVATE_P1 : [
        | after(1, sec)
        | ]
    Interruzione_LED_Verde_in_Chiuso_P1_Disattivo.DEACTIVATE_P1 -> Interruzione_LED_Verde_in_Chiuso_P1_Disattivo.VERIFY_DEACTIVATION : [
        | after(0.4, sec)
        | ]
    Interruzione_LED_Verde_in_Chiuso_P1_Disattivo.VERIFY_DEACTIVATION -> Interruzione_LED_Verde_in_Chiuso_P1_Disattivo.FINAL : [
        | after(1, sec)
        | ]
  state Interruzione_LED_Verde_in_Aperto_30_Secondi
    state INIT
      %% Initialize data outputs.
      p1 = true;
      p2 = false;
      start = false;
      b1 = false;
      b2 = false;
      b3 = false;
      verify(enable_green == false);
      verify(enable_yellow == false);
      verify(enable_red == false);
      verify(blink_green == false);
      verify(blink_yellow == false);
    state TURN_ON
      start = true;
    state CLOSE
      verify(enable_green == false);
      verify(enable_yellow == false);
      verify(enable_red == false);
      verify(blink_green == false);
      verify(blink_yellow == false);
    state PRESSED
      b1 = true;
    state RELEASED_BUTTON
      b1 = false;
    state OPENING_GATE
      p2 = true;
      verify(enable_green == false);
      verify(enable_yellow == false);
      verify(enable_red == false);
      verify(blink_green == false);
      verify(blink_yellow == true);
    state OPEN_GATE
      verify(enable_green == true);
      verify(enable_yellow == true);
      verify(enable_red == true);
      verify(blink_green == false);
      verify(blink_yellow == false);
    state ACTIVATE_P1
      p1 = false;
    state B1_PRESSED
      b1 = true;
    state B1_RELEASED_BUTTON
      b1 = false;
    state IGNORE_COMMAND
      verify(enable_green == false);
      verify(enable_yellow == false);
      verify(enable_red == false);
      verify(blink_green == true);
      verify(blink_yellow == false);
    state VERIFY_GREEN_LED
      verify(enable_green == false);
      verify(enable_yellow == false);
      verify(enable_red == false);
      verify(blink_green == true);
      verify(blink_yellow == false);
      settings: description=|
          | Stiamo verificando che
          | dopo 15 secondi il led
          | lampeggia ancora
          | in quanto p1 è ancora
          | attivo.
    state VERIFY_DEACTIVATION
      verify(enable_green == true);
      verify(enable_yellow == true);
      verify(enable_red == true);
      verify(blink_green == false);
      verify(blink_yellow == false);
      settings: description=|
          | Stiamo verificando che
          | dopo 30 secondi il led
          | si sia spento, come da
          | specifiche.
    state FINAL
      p2 = false;
    (default) -> Interruzione_LED_Verde_in_Aperto_30_Secondi.INIT
    Interruzione_LED_Verde_in_Aperto_30_Secondi.INIT -> Interruzione_LED_Verde_in_Aperto_30_Secondi.TURN_ON : [
        | after(2, sec)
        | ]
    Interruzione_LED_Verde_in_Aperto_30_Secondi.TURN_ON -> Interruzione_LED_Verde_in_Aperto_30_Secondi.CLOSE : [
        | after(3, sec)
        | ]
    Interruzione_LED_Verde_in_Aperto_30_Secondi.CLOSE -> Interruzione_LED_Verde_in_Aperto_30_Secondi.PRESSED : [
        | after(2, sec)
        | ]
    Interruzione_LED_Verde_in_Aperto_30_Secondi.PRESSED -> Interruzione_LED_Verde_in_Aperto_30_Secondi.RELEASED_BUTTON : [
        | after(2, sec)
        | ]
    Interruzione_LED_Verde_in_Aperto_30_Secondi.RELEASED_BUTTON -> Interruzione_LED_Verde_in_Aperto_30_Secondi.OPENING_GATE : [
        | after(0.4, sec)
        | ]
    Interruzione_LED_Verde_in_Aperto_30_Secondi.OPENING_GATE -> Interruzione_LED_Verde_in_Aperto_30_Secondi.OPEN_GATE : [
        | after(10, sec)
        | ]
    Interruzione_LED_Verde_in_Aperto_30_Secondi.OPEN_GATE -> Interruzione_LED_Verde_in_Aperto_30_Secondi.ACTIVATE_P1 : [
        | after(2, sec)
        | ]
    Interruzione_LED_Verde_in_Aperto_30_Secondi.ACTIVATE_P1 -> Interruzione_LED_Verde_in_Aperto_30_Secondi.B1_PRESSED : [
        | after(0.4, sec)
        | ]
    Interruzione_LED_Verde_in_Aperto_30_Secondi.B1_PRESSED -> Interruzione_LED_Verde_in_Aperto_30_Secondi.B1_RELEASED_BUTTON : [
        | after(2, sec)
        | ]
    Interruzione_LED_Verde_in_Aperto_30_Secondi.B1_RELEASED_BUTTON -> Interruzione_LED_Verde_in_Aperto_30_Secondi.IGNORE_COMMAND : [
        | after(0.4, sec)
        | ]
    Interruzione_LED_Verde_in_Aperto_30_Secondi.IGNORE_COMMAND -> Interruzione_LED_Verde_in_Aperto_30_Secondi.VERIFY_GREEN_LED : [
        | after(15, sec)
        | ]
    Interruzione_LED_Verde_in_Aperto_30_Secondi.VERIFY_GREEN_LED -> Interruzione_LED_Verde_in_Aperto_30_Secondi.VERIFY_DEACTIVATION : [
        | after(15, sec)
        | ]
    Interruzione_LED_Verde_in_Aperto_30_Secondi.VERIFY_DEACTIVATION -> Interruzione_LED_Verde_in_Aperto_30_Secondi.FINAL : [
        | after(1, sec)
        | ]
  state Interruzione_LED_Verde_in_Chiuso_30_Secondi
    state INIT
      %% Initialize data outputs.
      p1 = true;
      p2 = false;
      start = false;
      b1 = false;
      b2 = false;
      b3 = false;
      verify(enable_green == false);
      verify(enable_yellow == false);
      verify(enable_red == false);
      verify(blink_green == false);
      verify(blink_yellow == false);
    state TURN_ON
      start = true;
    state CLOSE
      verify(enable_green == false);
      verify(enable_yellow == false);
      verify(enable_red == false);
      verify(blink_green == false);
      verify(blink_yellow == false);
    state ACTIVATE_P1
      p1 = false;
    state PRESSED
      b1 = true;
    state RELEASED_BUTTON
      b1 = false;
    state IGNORE_COMMAND
      verify(enable_green == false);
      verify(enable_yellow == false);
      verify(enable_red == false);
      verify(blink_green == true);
      verify(blink_yellow == false);
    state VERIFY_GREEN_LED
      verify(enable_green == false);
      verify(enable_yellow == false);
      verify(enable_red == false);
      verify(blink_green == true);
      verify(blink_yellow == false);
    state VERIFY_DEACTIVATION
      verify(enable_green == false);
      verify(enable_yellow == false);
      verify(enable_red == false);
      verify(blink_green == false);
      verify(blink_yellow == false);
    state FINAL
    (default) -> Interruzione_LED_Verde_in_Chiuso_30_Secondi.INIT
    Interruzione_LED_Verde_in_Chiuso_30_Secondi.INIT -> Interruzione_LED_Verde_in_Chiuso_30_Secondi.TURN_ON : [
        | after(2, sec)
        | ]
    Interruzione_LED_Verde_in_Chiuso_30_Secondi.TURN_ON -> Interruzione_LED_Verde_in_Chiuso_30_Secondi.CLOSE : [
        | after(3, sec)
        | ]
    Interruzione_LED_Verde_in_Chiuso_30_Secondi.CLOSE -> Interruzione_LED_Verde_in_Chiuso_30_Secondi.ACTIVATE_P1 : [
        | after(2, sec)
        | ]
    Interruzione_LED_Verde_in_Chiuso_30_Secondi.ACTIVATE_P1 -> Interruzione_LED_Verde_in_Chiuso_30_Secondi.PRESSED : [
        | after(0.4, sec)
        | ]
    Interruzione_LED_Verde_in_Chiuso_30_Secondi.PRESSED -> Interruzione_LED_Verde_in_Chiuso_30_Secondi.RELEASED_BUTTON : [
        | after(2, sec)
        | ]
    Interruzione_LED_Verde_in_Chiuso_30_Secondi.RELEASED_BUTTON -> Interruzione_LED_Verde_in_Chiuso_30_Secondi.IGNORE_COMMAND : [
        | after(0.4, sec)
        | ]
    Interruzione_LED_Verde_in_Chiuso_30_Secondi.IGNORE_COMMAND -> Interruzione_LED_Verde_in_Chiuso_30_Secondi.VERIFY_GREEN_LED : [
        | after(15, sec)
        | ]
    Interruzione_LED_Verde_in_Chiuso_30_Secondi.VERIFY_DEACTIVATION -> Interruzione_LED_Verde_in_Chiuso_30_Secondi.FINAL : [
        | after(1, sec)
        | ]
    Interruzione_LED_Verde_in_Chiuso_30_Secondi.VERIFY_GREEN_LED -> Interruzione_LED_Verde_in_Chiuso_30_Secondi.VERIFY_DEACTIVATION : [
        | after(15, sec)
        | ]
  state Reset_Lampeggio_LED_Verde_in_Aperto
    state INIT
      %% Initialize data outputs.
      p1 = true;
      p2 = false;
      start = false;
      b1 = false;
      b2 = false;
      b3 = false;
      verify(enable_green == false);
      verify(enable_yellow == false);
      verify(enable_red == false);
      verify(blink_green == false);
      verify(blink_yellow == false);
    state TURN_ON
      start = true;
    state CLOSE
      verify(enable_green == false);
      verify(enable_yellow == false);
      verify(enable_red == false);
      verify(blink_green == false);
      verify(blink_yellow == false);
    state PRESSED
      b1 = true;
    state RELEASED_BUTTON
      b1 = false;
    state OPENING_GATE
      p2 = true;
      verify(enable_green == false);
      verify(enable_yellow == false);
      verify(enable_red == false);
      verify(blink_green == false);
      verify(blink_yellow == true);
    state OPEN_GATE
      verify(enable_green == true);
      verify(enable_yellow == true);
      verify(enable_red == true);
      verify(blink_green == false);
      verify(blink_yellow == false);
    state ACTIVATE_P1
      p1 = false;
    state B1_PRESSED
      b1 = true;
    state B1_RELEASED_BUTTON
      b1 = false;
    state IGNORE_COMMAND
      verify(enable_green == false);
      verify(enable_yellow == false);
      verify(enable_red == false);
      verify(blink_green == true);
      verify(blink_yellow == false);
    state B1_PRESSED_AGAIN
      b1 = true;
    state B1_RELEASED_BUTTON_AGAIN
      b1 = false;
      settings: description=|
          | La transizione
          | aspetta 15 secondi in
          | modo da far vedere
          | che passati 30 secondi
          | dalla prima accensione
          | del led esso non si
          | spegne, questo perché
          | il pulsante B1 è stato
          | premuto di nuovo.
    state VERIFY_GREEN_LED
      verify(enable_green == false);
      verify(enable_yellow == false);
      verify(enable_red == false);
      verify(blink_green == true);
      verify(blink_yellow == false);
      settings: description=|
          | Aspettiamo altri 15
          | secondi per raggiungere
          | 30 secondi dalla
          | seconda pressione di
          | B1, per verificare che
          | il led verde si sia spento
    state VERIFY_DEACTIVATION
      verify(enable_green == true);
      verify(enable_yellow == true);
      verify(enable_red == true);
      verify(blink_green == false);
      verify(blink_yellow == false);
    state FINAL
    (default) -> Reset_Lampeggio_LED_Verde_in_Aperto.INIT
    Reset_Lampeggio_LED_Verde_in_Aperto.INIT -> Reset_Lampeggio_LED_Verde_in_Aperto.TURN_ON : [
        | after(2, sec)
        | ]
    Reset_Lampeggio_LED_Verde_in_Aperto.TURN_ON -> Reset_Lampeggio_LED_Verde_in_Aperto.CLOSE : [
        | after(3, sec)
        | ]
    Reset_Lampeggio_LED_Verde_in_Aperto.CLOSE -> Reset_Lampeggio_LED_Verde_in_Aperto.PRESSED : [
        | after(2, sec)
        | ]
    Reset_Lampeggio_LED_Verde_in_Aperto.PRESSED -> Reset_Lampeggio_LED_Verde_in_Aperto.RELEASED_BUTTON : [
        | after(2, sec)
        | ]
    Reset_Lampeggio_LED_Verde_in_Aperto.RELEASED_BUTTON -> Reset_Lampeggio_LED_Verde_in_Aperto.OPENING_GATE : [
        | after(0.4, sec)
        | ]
    Reset_Lampeggio_LED_Verde_in_Aperto.OPENING_GATE -> Reset_Lampeggio_LED_Verde_in_Aperto.OPEN_GATE : [
        | after(10, sec)
        | ]
    Reset_Lampeggio_LED_Verde_in_Aperto.OPEN_GATE -> Reset_Lampeggio_LED_Verde_in_Aperto.ACTIVATE_P1 : [
        | after(2, sec)
        | ]
    Reset_Lampeggio_LED_Verde_in_Aperto.ACTIVATE_P1 -> Reset_Lampeggio_LED_Verde_in_Aperto.B1_PRESSED : [
        | after(0.4, sec)
        | ]
    Reset_Lampeggio_LED_Verde_in_Aperto.B1_PRESSED -> Reset_Lampeggio_LED_Verde_in_Aperto.B1_RELEASED_BUTTON : [
        | after(2, sec)
        | ]
    Reset_Lampeggio_LED_Verde_in_Aperto.B1_RELEASED_BUTTON -> Reset_Lampeggio_LED_Verde_in_Aperto.IGNORE_COMMAND : [
        | after(0.4, sec)
        | ]
    Reset_Lampeggio_LED_Verde_in_Aperto.IGNORE_COMMAND -> Reset_Lampeggio_LED_Verde_in_Aperto.B1_PRESSED_AGAIN : [
        | after(15, sec)
        | ]
    Reset_Lampeggio_LED_Verde_in_Aperto.VERIFY_GREEN_LED -> Reset_Lampeggio_LED_Verde_in_Aperto.VERIFY_DEACTIVATION : [
        | after(15.4, sec)
        | ]
    Reset_Lampeggio_LED_Verde_in_Aperto.VERIFY_DEACTIVATION -> Reset_Lampeggio_LED_Verde_in_Aperto.FINAL : [
        | after(5, sec)
        | ]
    Reset_Lampeggio_LED_Verde_in_Aperto.B1_PRESSED_AGAIN -> Reset_Lampeggio_LED_Verde_in_Aperto.B1_RELEASED_BUTTON_AGAIN : [
        | after(2, sec)
        | ]
    Reset_Lampeggio_LED_Verde_in_Aperto.B1_RELEASED_BUTTON_AGAIN -> Reset_Lampeggio_LED_Verde_in_Aperto.VERIFY_GREEN_LED : [
        | after(15, sec)
        | ]
  state Reset_Lampeggio_LED_Verde_in_Chiuso
    state INIT
      %% Initialize data outputs.
      p1 = true;
      p2 = false;
      start = false;
      b1 = false;
      b2 = false;
      b3 = false;
      verify(enable_green == false);
      verify(enable_yellow == false);
      verify(enable_red == false);
      verify(blink_green == false);
      verify(blink_yellow == false);
    state TURN_ON
      start = true;
    state CLOSE
      verify(enable_green == false);
      verify(enable_yellow == false);
      verify(enable_red == false);
      verify(blink_green == false);
      verify(blink_yellow == false);
    state ACTIVATE_P1
      p1 = false;
    state PRESSED
      b1 = true;
    state RELEASED_BUTTON
      b1 = false;
    state IGNORE_COMMAND
      verify(enable_green == false);
      verify(enable_yellow == false);
      verify(enable_red == false);
      verify(blink_green == true);
      verify(blink_yellow == false);
    state B1_PRESSED_AGAIN
      b1 = true;
    state B1_RELEASED_BUTTON_AGAIN
      b1 = false;
      settings: description=|
          | La transizione
          | aspetta 15 secondi in
          | modo da far vedere
          | che passati 30 secondi
          | dalla prima accensione
          | del led esso non si
          | spegne, questo perché
          | il pulsante B1 è stato
          | premuto di nuovo.
    state VERIFY_GREEN_LED
      verify(enable_green == false);
      verify(enable_yellow == false);
      verify(enable_red == false);
      verify(blink_green == true);
      verify(blink_yellow == false);
      settings: description=|
          | Aspettiamo altri 15
          | secondi per raggiungere
          | 30 secondi dalla
          | seconda pressione di
          | B1, per verificare che
          | il led verde si sia spento
    state VERIFY_DEACTIVATION
      verify(enable_green == false);
      verify(enable_yellow == false);
      verify(enable_red == false);
      verify(blink_green == false);
      verify(blink_yellow == false);
    state FINAL
    (default) -> Reset_Lampeggio_LED_Verde_in_Chiuso.INIT
    Reset_Lampeggio_LED_Verde_in_Chiuso.INIT -> Reset_Lampeggio_LED_Verde_in_Chiuso.TURN_ON : [
        | after(2, sec)
        | ]
    Reset_Lampeggio_LED_Verde_in_Chiuso.TURN_ON -> Reset_Lampeggio_LED_Verde_in_Chiuso.CLOSE : [
        | after(3, sec)
        | ]
    Reset_Lampeggio_LED_Verde_in_Chiuso.CLOSE -> Reset_Lampeggio_LED_Verde_in_Chiuso.ACTIVATE_P1 : [
        | after(2, sec)
        | ]
    Reset_Lampeggio_LED_Verde_in_Chiuso.PRESSED -> Reset_Lampeggio_LED_Verde_in_Chiuso.RELEASED_BUTTON : [
        | after(2, sec)
        | ]
    Reset_Lampeggio_LED_Verde_in_Chiuso.IGNORE_COMMAND -> Reset_Lampeggio_LED_Verde_in_Chiuso.B1_PRESSED_AGAIN : [
        | after(15, sec)
        | ]
    Reset_Lampeggio_LED_Verde_in_Chiuso.B1_PRESSED_AGAIN -> Reset_Lampeggio_LED_Verde_in_Chiuso.B1_RELEASED_BUTTON_AGAIN : [
        | after(2, sec)
        | ]
    Reset_Lampeggio_LED_Verde_in_Chiuso.B1_RELEASED_BUTTON_AGAIN -> Reset_Lampeggio_LED_Verde_in_Chiuso.VERIFY_GREEN_LED : [
        | after(15, sec)
        | ]
    Reset_Lampeggio_LED_Verde_in_Chiuso.VERIFY_GREEN_LED -> Reset_Lampeggio_LED_Verde_in_Chiuso.VERIFY_DEACTIVATION : [
        | after(15.4, sec)
        | ]
    Reset_Lampeggio_LED_Verde_in_Chiuso.VERIFY_DEACTIVATION -> Reset_Lampeggio_LED_Verde_in_Chiuso.FINAL : [
        | after(5, sec)
        | ]
    Reset_Lampeggio_LED_Verde_in_Chiuso.ACTIVATE_P1 -> Reset_Lampeggio_LED_Verde_in_Chiuso.PRESSED : [
        | after(0.4, sec)
        | ]
    Reset_Lampeggio_LED_Verde_in_Chiuso.RELEASED_BUTTON -> Reset_Lampeggio_LED_Verde_in_Chiuso.IGNORE_COMMAND : [
        | after(0.4, sec)
        | ]
  (default) -> Apertura_Chiusura_con_B1 [order 1] : [Active_Scenario_Index == 1]
  (default) -> Chiusura_Automatica [order 2] : [Active_Scenario_Index == 2]
  (default) -> Richiesta_Chiusura_durante_Apertura [order 3] : [Active_Scenario_Index == 3]
  (default) -> Richiesta_Apertura_durante_Chiusura [order 4] : [Active_Scenario_Index == 4]
  (default) -> Incremento_Tempo_Lavoro [order 5] : [Active_Scenario_Index == 5]
  (default) -> Incremento_Tempo_Chiusura_Automatica [order 6] : [Active_Scenario_Index == 6]
  (default) -> Gestione_Situazione_Errore [order 7] : [Active_Scenario_Index == 7]
  (default) -> Stato_di_Blocco [order 8] : [Active_Scenario_Index == 8]
  (default) -> Stato_di_Errore [order 9] : [Active_Scenario_Index == 9]
  (default) -> Rilevamento_Ostacolo_in_Chiusura [order 10] : [Active_Scenario_Index == 10]
  (default) -> RIlevamento_Ostacolo_in_Apertura [order 11] : [Active_Scenario_Index == 11]
  (default) -> Interruzione_Tempo_Chiusura_Automatica_con_Ostacoli [order 12] : [Active_Scenario_Index == 12]
  (default) -> Interruzione_LED_Verde_in_Aperto_P1_Disattivo [order 13] : [Active_Scenario_Index == 13]
  (default) -> Interruzione_LED_Verde_in_Chiuso_P1_Disattivo [order 14] : [Active_Scenario_Index == 14]
  (default) -> Interruzione_LED_Verde_in_Aperto_30_Secondi [order 15] : [Active_Scenario_Index == 15]
  (default) -> Interruzione_LED_Verde_in_Chiuso_30_Secondi [order 16] : [Active_Scenario_Index == 16]
  (default) -> Reset_Lampeggio_LED_Verde_in_Aperto [order 17] : [Active_Scenario_Index == 17]
  (default) -> Reset_Lampeggio_LED_Verde_in_Chiuso [order 18] : {assert(Active_Scenario_Index == 18,'The value of Scenario Parameter ''Active_Scenario_Index'' is not valid. Use the index of the scenario to specify it.')}
  data: enable_green input boolean size=[1]; blink_green input boolean size=[1]; enable_red input boolean size=[1]; enable_yellow input boolean size=[1]; blink_yellow input boolean size=[1]; p1 output boolean size=[1]; p2 output boolean size=[1]; start output boolean size=[1]; b1 output boolean size=[1]; b2 output boolean size=[1]; b3 output boolean size=[1]; Active_Scenario_Index parameter =18; n local; MAX constant double =120; INCREMENT constant double =10
